simulink subsystem "PieroAdry_MODELZ"  (R2023b)
settings: Solver=VariableStepAuto  StartTime=0.0  StopTime=10.0  RelTol=1e-3
settings Model: Creator=adria  LastModifiedBy=adria

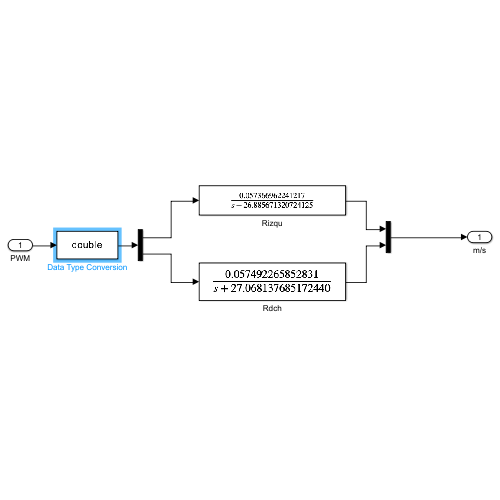
[thumbnail: Simulink's stored preview of the top-level diagram]
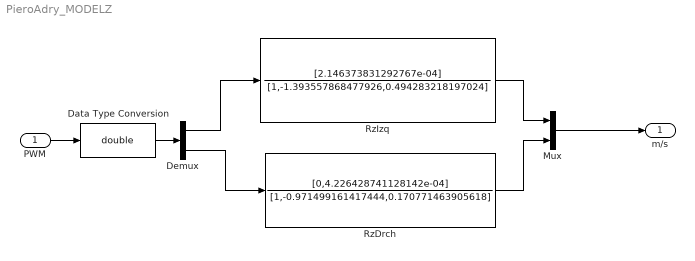
== system PieroAdry_MODELZ ==
  PWM : Inport
  Data Type Conversion : DataTypeConversion  OutDataTypeStr=double  SaturateOnIntegerOverflow=off  RndMeth=Floor
  Demux : Demux  Outputs=2
  Mux : Mux  Inputs=2
  RzDrch : DiscreteFilter  Numerator=[0,4.226428741128142e-04]  Denominator=[1,-0.971499161417444,0.170771463905618]
  RzIzq : DiscreteFilter  Numerator=[2.146373831292767e-04]  Denominator=[1,-1.393557868477926,0.494283218197024]
  m/s : Outport
  wires:
  RzIzq/1 -> Mux/1
  PWM/1 -> Data Type Conversion/1
  Demux/1 -> RzIzq/1
  Demux/2 -> RzDrch/1
  Mux/1 -> m/s/1
  RzDrch/1 -> Mux/2
  Data Type Conversion/1 -> Demux/1
